simulink model "frek_test_sim"  (Simulink 8.0)
settings: Solver=ode1  SolverMode=SingleTasking  StartTime=0.0  StopTime=5  FixedStep=0.001  RelTol=1e-3
values from neighbouring files (symbols this model uses):
  Beq = 0.0015*6    (= 0.009)    [Sve ikad.m]    (also in matlab.mat = 0.0075)
  den_k = [1 100*a]    [Sve ikad.m]    (also in matlab.mat = [1 286.356023126])
  Eff_G = 0.9    [Sve ikad.m]    (also in matlab.mat)
  Eff_M = 0.69    [Sve ikad.m]    (also in matlab.mat)
  Jeq = 2e-3    (= 0.002)    [Sve ikad.m]    (also in matlab.mat)
  Ke = 0.0076776    [Sve ikad.m]    (also in matlab.mat)
  Kg = 70    [Sve ikad.m]    (also in matlab.mat)
  Km = 0.007683    [Sve ikad.m]    (also in matlab.mat)
  Kp = 41.5    [Sve ikad.m]    (also in matlab.mat = 160)
  num_k = [1*a 100]    [Sve ikad.m]    (also in matlab.mat = [2.86356023126 100])
  Ra = 2.6    [Sve ikad.m]    (also in matlab.mat)
settings Model: Creator=Niko  LastModifiedBy=Niko

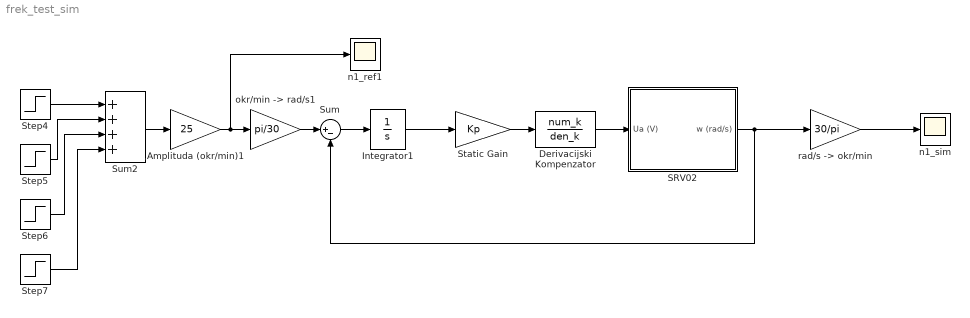
== system frek_test_sim ==
  Amplituda (okr/min)1 : Gain  Gain=25
  Derivacijski Kompenzator : TransferFcn  Numerator=num_k  Denominator=den_k
  Integrator1 : Integrator
  "SRV02 " : Subsystem
  Static Gain : Gain  Gain=Kp
  Step4 : Step  Time=1.015
  Step5 : Step  Time=1.03  After=-1
  Step6 : Step  Time=1.045  After=-1
  Step7 : Step  Time=1.06
  Sum : Sum  Inputs=|+-
  Sum2 : Sum  Inputs=++++
  n1_ref1 : Scope
      settings: TimeRange=5  YMin=0  YMax=30  SaveName=n_opt  SampleInput=on
  n1_sim : Scope
      settings: TimeRange=5  YMin=0  YMax=30  SaveName=n_sim_opt  SampleInput=on
  "okr/min -> rad/s1" : Gain  Gain=pi/30
  "rad/s -> okr/min" : Gain  Gain=30/pi
  wires:
  Static Gain/1 -> Derivacijski Kompenzator/1
  Sum/1 -> Integrator1/1
  Integrator1/1 -> Static Gain/1
  Derivacijski Kompenzator/1 -> "SRV02 "/1(Ua (V))
  "SRV02 "/1(w (rad/s)) -> Sum/2, "rad/s -> okr/min"/1
  "rad/s -> okr/min"/1 -> n1_sim/1
  Amplituda (okr/min)1/1 -> "okr/min -> rad/s1"/1, n1_ref1/1
  Sum2/1 -> Amplituda (okr/min)1/1
  Step7/1 -> Sum2/4
  Step6/1 -> Sum2/3
  Step5/1 -> Sum2/2
  Step4/1 -> Sum2/1
  "okr/min -> rad/s1"/1 -> Sum/1

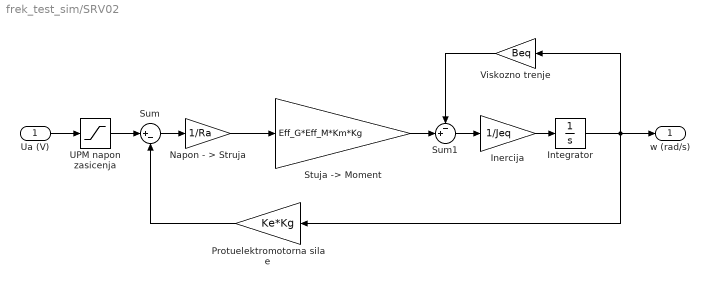
== system frek_test_sim/SRV02  ==
  Ua (V) : Inport
  Inercija : Gain  Gain=1/Jeq
  Integrator : Integrator
  Napon - > Struja : Gain  Gain=1/Ra
  Protuelektromotorna sila e : Gain  Gain=Ke*Kg
  "Stuja -> Moment" : Gain  Gain=Eff_G*Eff_M*Km*Kg
  Sum : Sum  Inputs=|+-
  Sum1 : Sum  Inputs=-+|
  UPM napon zasicenja : Saturate  UpperLimit=6  LowerLimit=-6
  Viskozno trenje : Gain  Gain=Beq
  w (rad/s) : Outport
  wires:
  Sum1/1 -> Inercija/1
  "Stuja -> Moment"/1 -> Sum1/2
  Inercija/1 -> Integrator/1
  UPM napon zasicenja/1 -> Sum/1
  Napon - > Struja/1 -> "Stuja -> Moment"/1
  Ua (V)/1 -> UPM napon zasicenja/1
  Sum/1 -> Napon - > Struja/1
  Viskozno trenje/1 -> Sum1/1
  Protuelektromotorna sila e/1 -> Sum/2
  Integrator/1 -> w (rad/s)/1, Protuelektromotorna sila e/1, Viskozno trenje/1
